simulink model "stateflow_logic"  (R2024b)
settings: Solver=VariableStepAuto  StartTime=0.0  StopTime=10  RelTol=1e-3
settings Model: Creator=abdur  LastModifiedBy=abdur

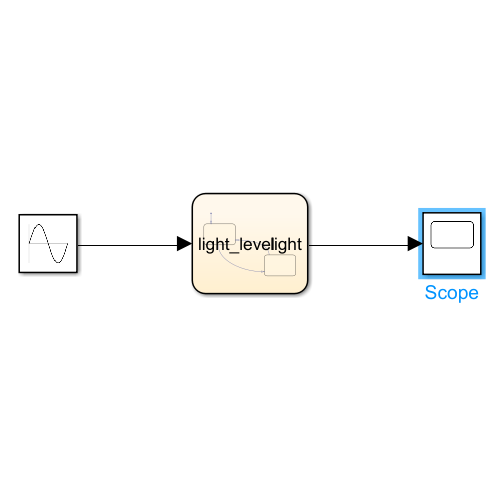
[thumbnail: Simulink's stored preview of the top-level diagram]
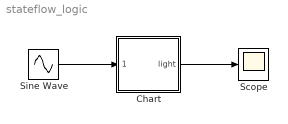
== system stateflow_logic ==
  Chart : Stateflow chart  TreatAsAtomicUnit=on
  Scope : Scope
  Sine Wave : Sin  Amplitude=20  Bias=30  SampleTime=0
  wires:
  Sine Wave/1 -> Chart/1(light_level)
  Chart/1(light) -> Scope/1

== stateflow chart stateflow_logic/Chart ==
  state Daytime
    light = 0;
  state Nighttime
    light = 1;
  (default) -> Daytime
  Nighttime -> Daytime : [light_level >  30]
  Daytime -> Nighttime : [light_level <= 30]
  data: light_level input double; light output double
